simulink model "FPGA_Comm_adc_dac"  (Simulink 7.6)
settings: Solver=ode4  StartTime=0.0  StopTime=500  FixedStep=0.01  MaxStep=1e-1  RelTol=1e-3
settings Model: Creator=jordan  LastModifiedBy=jordan
settings GRTTargetCC: ExtMode=on

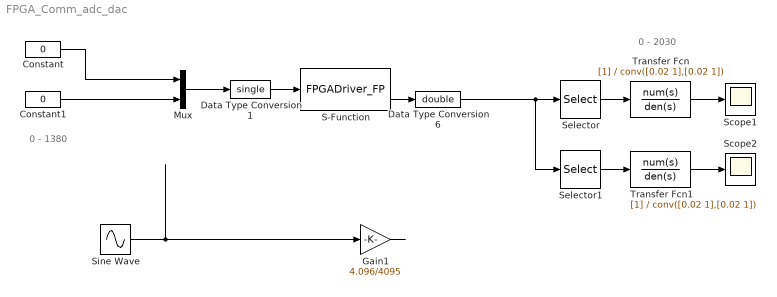
== system FPGA_Comm_adc_dac ==
  note: 0 - 1380
  note: 0 - 2030
  Constant : Constant  Value=0
  Constant1 : Constant  Value=0
  Data Type Conversion1 : DataTypeConversion  OutDataTypeStr=single
  Data Type Conversion6 : DataTypeConversion  OutDataTypeStr=double
  Gain1 : Gain  Gain=4.096/4095
  Mux : Mux  Inputs=2
  S-Function : S-Function  FunctionName=FPGADriver_FP  EnableBusSupport=off
  Scope1 : Scope
      settings: TimeRange=50  YMin=1200  YMax=2900  MaxDataPoints=50000
  Scope2 : Scope
      settings: TimeRange=50  YMin=1380  YMax=1470  MaxDataPoints=50000
  Selector : Selector  InputPortWidth=4  IndexOptions=Index vector (dialog)  Indices=1  OutputSizes=1
  Selector1 : Selector  InputPortWidth=4  IndexOptions=Index vector (dialog)  Indices=2  OutputSizes=1
  Sine Wave : Sin  Amplitude=1000  Bias=1000  Frequency=2*pi  SampleTime=0
  Transfer Fcn : TransferFcn  Denominator=conv([0.02 1],[0.02 1])
  Transfer Fcn1 : TransferFcn  Denominator=conv([0.02 1],[0.02 1])
  wires:
  S-Function/2 -> Data Type Conversion6/1
  Data Type Conversion1/1 -> S-Function/1
  Data Type Conversion6/1 -> Selector/1, Selector1/1
  Mux/1 -> Data Type Conversion1/1
  Selector/1 -> Transfer Fcn/1
  Selector1/1 -> Transfer Fcn1/1
  Constant1/1 -> Mux/2
  Sine Wave/1 -> Gain1/1
  Gain1/1 -> ?
  Constant/1 -> Mux/1
  Transfer Fcn/1 -> Scope1/1
  Transfer Fcn1/1 -> Scope2/1
